simulink subsystem "MB"  (R2023a)
settings: Solver=VariableStepAuto  StartTime=0.0  StopTime=10.0  RelTol=1e-3
values from neighbouring files (symbols this model uses):
  d = 7.9379e-12    [constants.m]
  k = 3.1582e-10    [constants.m]
  l = 39.73e-3    (= 0.03973)    [constants.m]
settings Model: Creator=raphb  LastModifiedBy=raphb

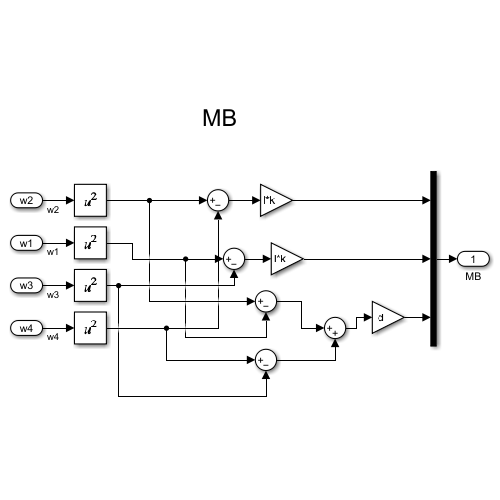
[thumbnail: Simulink's stored preview of the top-level diagram]
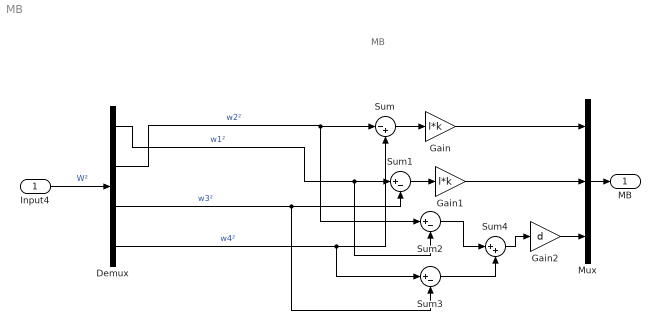
== system MB ==
  note: MB
  Input4 : Inport
  Demux : Demux
  Gain : Gain  Gain=l*k
  Gain1 : Gain  Gain=l*k
  Gain2 : Gain  Gain=d
  Mux : Mux  Inputs=3
  Sum : Sum  Inputs=|-+
  Sum1 : Sum  Inputs=|+-
  Sum2 : Sum  Inputs=|+-
  Sum3 : Sum  Inputs=|+-
  Sum4 : Sum  Inputs=|++
  MB : Outport
  wires:
  Demux/2 -> Sum2/1, Sum/1  "w2²"
  Demux/4 -> Sum3/1, Sum/2  "w4²"
  Sum/1 -> Gain/1
  Gain/1 -> Mux/1
  Sum2/1 -> Sum4/1
  Gain2/1 -> Mux/3
  Mux/1 -> MB/1
  Demux/1 -> Sum2/2, Sum1/1  "w1²"
  Demux/3 -> Sum3/2, Sum1/2  "w3²"
  Sum3/1 -> Sum4/2
  Gain1/1 -> Mux/2
  Sum1/1 -> Gain1/1
  Sum4/1 -> Gain2/1
  Input4/1 -> Demux/1  "W²"
